simulink model "plsworkkkkk"  (R2023b)
settings: Solver=ode8  StartTime=0.0  StopTime=10.0  FixedStep=0.01  RelTol=1e-3
values from neighbouring files (symbols this model uses):
  g = 9.81    [Cube.m]    (also in parameters.m)
  gamma = [1 1 -1 0; 1 -1 0 1; -1 0 -1 1; 0 1 1 1]    [Cube.m]    (also in parameters.m)
  Ic_bar = (IcO - Iw)    [parameters.m]    (also in paramters.m = IcO - Iw)
  invIc_bar = inv(Ic_bar)    [parameters.m]
  invIw = inv(Iw)    [parameters.m]
  Iw = [Iwxx 0 0; 0 Iwxx 0; 0 0 Iwxx]    [parameters.m]    (also in paramters.m; reaction_wheel_params.m)
  l = 0.15    [parameters.m]    (also in paramters.m)
  mc_bar = ms + 2*mw    [Cube.m]    (also in parameters.m = 0.74)
  qr = [sqrt((2/3) * (3 + sqrt(3)))/2; sqrt((1/3) * (3 - sqrt(3)))/2; -sqrt((1/3) * (3 - sqrt(3)))/2; 0]    [parameters.m]
  wr = [0;0;0;0]    [parameters.m]
  wrdot = [0;0;0;0]    [parameters.m]
libraries: aerolibutil x7, matrix_library x3, sharedutil x1, vrlib x1
settings Model: Creator=kriti  LastModifiedBy=kriti
settings DebuggingCC: SolverPrmCheckMsg=warning  StateNameClashWarn=warning

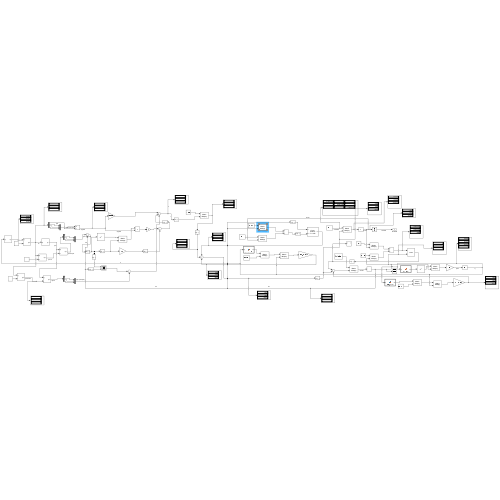
[thumbnail: Simulink's stored preview of the top-level diagram]
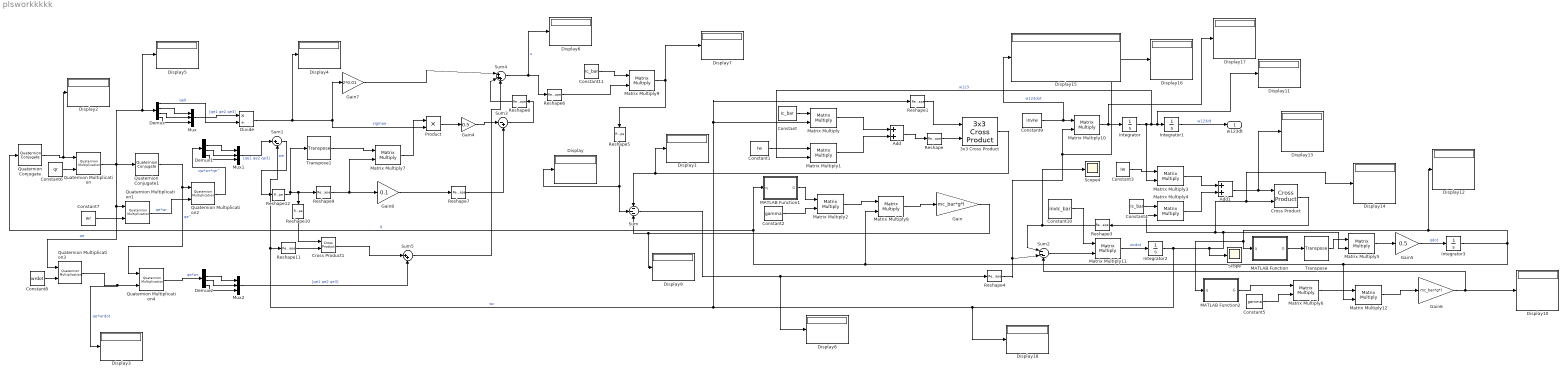
== system plsworkkkkk ==
  3x3 Cross Product : sharedutil/3x3 Cross Product  aMode=aMode
      settings: LibrarySourceBlock=aerolibutil/3x3 Cross Product
  Add : Sum
  Add1 : Sum
  Constant : Constant  Value=Ic_bar  VectorParams1D=off
  Constant1 : Constant  Value=Iw
  Constant10 : Constant  Value=invIc_bar  VectorParams1D=off
  Constant11 : Constant  Value=Ic_bar
  Constant2 : Constant  Value=gamma
  Constant3 : Constant  Value=Iw
  Constant4 : Constant  Value=Ic_bar
  Constant5 : Constant  Value=gamma
  Constant6 : Constant  Value=qr
  Constant7 : Constant  Value=wr
  Constant8 : Constant  Value=wrdot
  Constant9 : Constant  Value=invIw  VectorParams1D=off
  Cross Product : matrix_library/Cross Product
  Cross Product1 : vrlib/Utilities/Cross Product
  Demux : Demux
  Demux1 : Demux
  Demux2 : Demux
  Display{,1..18} (19 alike) : Display
  Divide : Product  Inputs=*/
  Gain : Gain  Gain=mc_bar*g*l
  Gain4 : Gain  Gain=0.5
  Gain5 : Gain  Gain=0.5
  Gain6 : Gain  Gain=mc_bar*g*l
  Gain7 : Gain  Gain=2*0.01
  Gain8 : Gain  Gain=0.1
  Integrator : Integrator
  Integrator1 : Integrator
  Integrator2 : Integrator
  Integrator3 : Integrator  InitialCondition=[sqrt((2/3) * (3 + sqrt(3)))/2; sqrt((1/3) * (3 - sqrt(3)))/2; -sqrt((1/3) * (3 - sqrt(3)))/2; 0]
  MATLAB Function : MATLAB Function  TreatAsAtomicUnit=on
  MATLAB Function1 : MATLAB Function  TreatAsAtomicUnit=on
  MATLAB Function2 : MATLAB Function  TreatAsAtomicUnit=on
  Matrix Multiply{,1..12} (13 alike) : Product  Multiplication=Matrix(*)
  Mux : Mux  Inputs=3
  Mux1 : Mux  Inputs=3
  Mux2 : Mux  Inputs=3
  Product : Product
  Quaternion Conjugate : aerolibutil/Quaternion Conjugate
  Quaternion Conjugate1 : aerolibutil/Quaternion Conjugate
  Quaternion Multiplication{,1..4} (5 alike) : aerolibutil/Quaternion Multiplication
  Reshape{,1,3..12} (12 alike) : Reshape
  Scope : Scope
  Scope4 : Scope
  Sum : Sum  Inputs=---
  Sum1 : Sum  Inputs=|+-
  Sum2 : Sum  Inputs=|---
  Sum3 : Sum  Inputs=|-+
  Sum4 : Sum  Inputs=|+++
  Sum5 : Sum  Inputs=|++
  Transpose : matrix_library/Transpose
  Transpose1 : matrix_library/Transpose
  w123dt : Outport
  wires:
  Constant/1 -> Matrix Multiply/1
  3x3 Cross Product/1 -> Display1/1, Sum/1
  Sum4/1 -> Display6/1, Reshape6/1  "u"
  Gain/1 -> Display9/1, Sum/3
  Matrix Multiply/1 -> Add/1
  Matrix Multiply1/1 -> Add/2
  MATLAB Function1/1(G) -> Matrix Multiply2/1
  Constant2/1 -> Matrix Multiply2/2
  MATLAB Function/1(G) -> Transpose/1
  Matrix Multiply5/1 -> Gain5/1
  Matrix Multiply4/1 -> Add1/2
  Gain5/1 -> Integrator3/1  "qdot"
  Integrator1/1 -> w123dt/1  "w123dt"
  Constant3/1 -> Matrix Multiply3/1
  Matrix Multiply3/1 -> Add1/1
  Constant4/1 -> Matrix Multiply4/1
  Matrix Multiply11/1 -> Integrator2/1  "wcdot"
  Gain6/1 -> Sum2/3, Display10/1
  Integrator2/1 -> Scope/1, Matrix Multiply5/2, Display14/1, Cross Product/2, Matrix Multiply4/2, Display18/1, Sum1/2, Reshape11/1, Matrix Multiply/2, Reshape1/1  "wc"
  Integrator/1 -> Matrix Multiply3/2, Matrix Multiply1/2, Display11/1, Integrator1/1  "w123"
  Sum/1 -> Display8/1, Reshape4/1
  Constant5/1 -> Matrix Multiply6/2
  MATLAB Function2/1(G) -> Matrix Multiply6/1
  Integrator3/1 -> Matrix Multiply12/2, Matrix Multiply8/2, Quaternion Conjugate/1, MATLAB Function1/1(q), Display12/1, MATLAB Function2/1(q), MATLAB Function/1(q)  "q"
  Cross Product/1 -> Reshape3/1
  Add1/1 -> Display13/1, Cross Product/1
  Sum2/1 -> Matrix Multiply11/2
  Demux/3 -> Mux/2
  Constant8/1 -> Quaternion Multiplication3/2
  Sum5/1 -> Sum4/3
  Quaternion Conjugate/1 -> Display2/1, Quaternion Multiplication/1
  Sum1/1 -> Reshape12/1  "we"
  Demux/1 -> Divide/2  "qe0"
  Demux/2 -> Mux/1
  Product/1 -> Gain4/1
  Transpose1/1 -> Matrix Multiply7/1
  Cross Product1/1 -> Sum5/1
  Mux/1 -> Divide/1  "[qe1 qe2 qe3]"
  Demux/4 -> Mux/3
  Constant7/1 -> Quaternion Multiplication1/2
  Gain8/1 -> Reshape7/1
  Gain4/1 -> Sum3/1
  Divide/1 -> Display4/1, Product/2, Gain7/1  "sigmae"
  Constant6/1 -> Quaternion Multiplication/2
  Sum3/1 -> Reshape8/1
  Quaternion Multiplication1/1 -> Quaternion Multiplication2/2  "qe*wr"
  Quaternion Multiplication3/1 -> Display3/1, Quaternion Multiplication4/2  "qe*wrdot"
  Gain7/1 -> Sum4/1
  Matrix Multiply7/1 -> Product/1
  Quaternion Multiplication/1 -> Display5/1, Demux/1, Quaternion Multiplication3/1, Quaternion Multiplication1/1, Quaternion Conjugate1/1  "qe"
  Quaternion Conjugate1/1 -> Quaternion Multiplication4/1, Quaternion Multiplication2/1  "qe^"
  Matrix Multiply9/1 -> Reshape5/1, Display7/1
  Matrix Multiply10/1 -> Display17/1, Integrator/1
  Constant9/1 -> Display15/1, Matrix Multiply10/1  "w123dot"
  Constant10/1 -> Matrix Multiply11/1
  Add/1 -> Reshape/1
  Reshape/1 -> 3x3 Cross Product/2
  Reshape1/1 -> 3x3 Cross Product/1
  Reshape4/1 -> Display16/1, Matrix Multiply10/2, Sum2/2
  Reshape3/1 -> Scope4/1, Sum2/1
  Reshape5/1 -> Display/1, Sum/2
  Reshape6/1 -> Matrix Multiply9/2
  Reshape7/1 -> Sum3/2
  Reshape8/1 -> Sum4/2
  Reshape9/1 -> Matrix Multiply7/2, Gain8/1
  Reshape10/1 -> Cross Product1/1
  Reshape11/1 -> Cross Product1/2
  Reshape12/1 -> Transpose1/1, Reshape9/1, Reshape10/1
  Constant1/1 -> Matrix Multiply1/1
  Matrix Multiply2/1 -> Matrix Multiply8/1
  Matrix Multiply8/1 -> Gain/1
  Matrix Multiply6/1 -> Matrix Multiply12/1
  Matrix Multiply12/1 -> Gain6/1
  Transpose/1 -> Matrix Multiply5/1
  Demux1/2 -> Mux1/1
  Demux1/4 -> Mux1/3
  Mux1/1 -> Sum1/1  "[qe1 qe2 qe3]"
  Demux1/3 -> Mux1/2
  Quaternion Multiplication2/1 -> Demux1/1  "qw*wr*qe^"
  Demux2/2 -> Mux2/1
  Demux2/4 -> Mux2/3
  Mux2/1 -> Sum5/2  "[qe1 qe2 qe3]"
  Demux2/3 -> Mux2/2
  Quaternion Multiplication4/1 -> Demux2/1  "qe*wr"
  Constant11/1 -> Matrix Multiply9/1

== matlab function plsworkkkkk/MATLAB Function ==
  data: q input; G output
function G = computeG(q)
    q0 = q(1); q1 = q(2); q2 = q(3); q3 = q(4);
    q_vector = [q1; q2; q3];
    q_skew = [0 -q3 q2; q3 0 -q1; q2 q1 0];
    G = [q_vector q0*eye(3) - q_skew];
end

== matlab function plsworkkkkk/MATLAB Function1 ==
  data: q input; G output
function G = computeG(q)
    q0 = q(1); q1 = q(2); q2 = q(3); q3 = q(4);
    q_vector = [q1; q2; q3];
    q_skew = [0 -q3 q2; q3 0 -q1; q2 q1 0];
    G = [q_vector q0*eye(3) - q_skew];
end

== matlab function plsworkkkkk/MATLAB Function2 ==
  data: q input; G output
function G = computeG(q)
    q0 = q(1); q1 = q(2); q2 = q(3); q3 = q(4);
    q_vector = [q1; q2; q3];
    q_skew = [0 -q3 q2; q3 0 -q1; q2 q1 0];
    G = [q_vector q0*eye(3) - q_skew];
end
